simulink model "ce4951txrcv"  (R2020b)
settings: Solver=VariableStepAuto  StartTime=0.0  StopTime=32  RelTol=1e-3
libraries: simulink_extras x11, dspsrcs4 x1
settings Model: Creator=Andy  LastModifiedBy=Andy

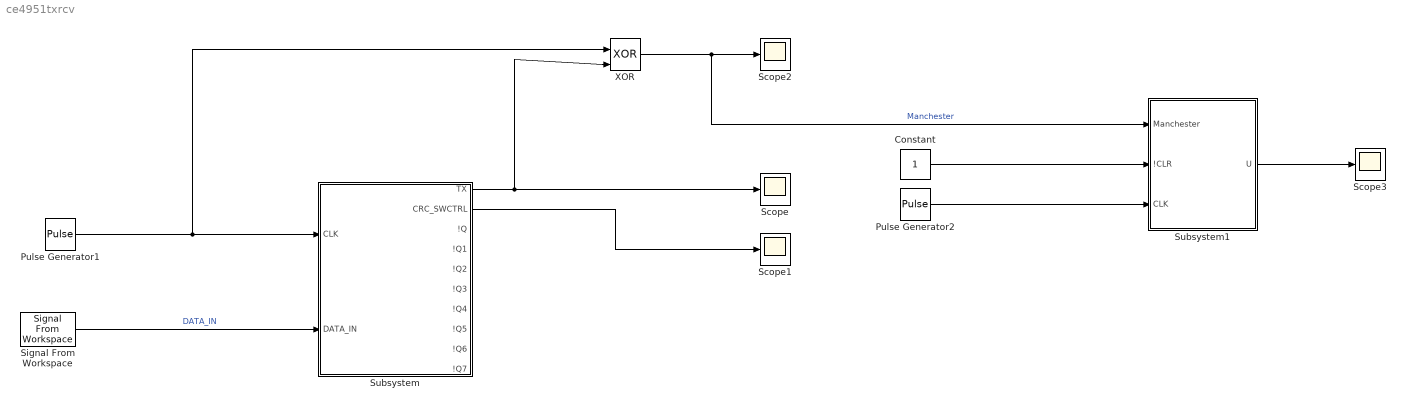
== system ce4951txrcv ==
  Constant : Constant
  Pulse Generator1 : DiscretePulseGenerator  PulseType=Time based  Period=1  PulseWidth=50
  Pulse Generator2 : DiscretePulseGenerator  PulseType=Time based  Period=0.5  PulseWidth=50
  Scope{,1..3} (4 alike) : Scope
  Signal From Workspace : dspsrcs4/Signal From Workspace  X=[0 1 0 0 0 0 0 1 0 1 0 0 0 0 1 0 0 1 0 0 0 0 1 1 0 0 0 0 0 0 0 0]  Ts=1  nsamps=1  OutputAfterFinalValue=Setting to zero  ignoreOrWarnInputAndFrameLengths=off  OutputFrames=off
  Subsystem : Subsystem
  Subsystem1 : Subsystem
  XOR : Logic  Operator=XOR  IconShape=distinctive  AllPortsSameDT=off  OutDataTypeStr=boolean
  wires:
  Subsystem/2(CRC_SWCTRL) -> Scope1/1
  XOR/1 -> Subsystem1/1(Manchester), Scope2/1  "Manchester"
  Signal From Workspace/1 -> Subsystem/2(DATA_IN)  "DATA_IN"
  Subsystem/1(TX) -> XOR/2, Scope/1
  Pulse Generator1/1 -> XOR/1, Subsystem/1(CLK)
  Pulse Generator2/1 -> Subsystem1/3(CLK)
  Constant/1 -> Subsystem1/2(!CLR)
  Subsystem1/1(U) -> Scope3/1

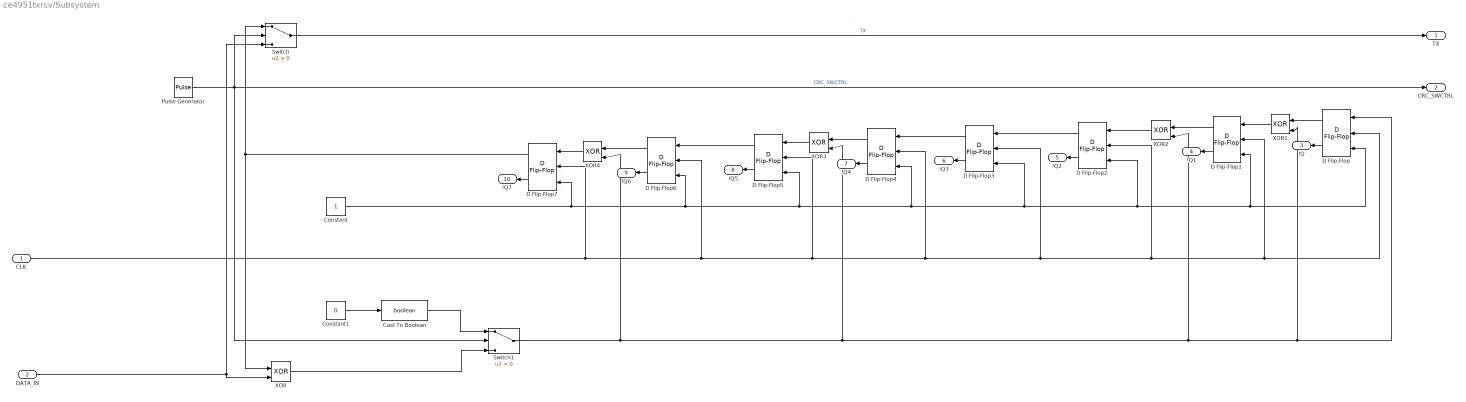
== system ce4951txrcv/Subsystem ==
  CLK : Inport
  DATA_IN : Inport  Port=2
  Cast To Boolean : DataTypeConversion  OutDataTypeStr=boolean
  Constant : Constant
  Constant1 : Constant  Value=0
  D Flip-Flop{,1..7} (8 alike) : simulink_extras/Flip Flops/D Flip-Flop
  Pulse Generator : DiscretePulseGenerator  PulseType=Time based  Period=32  PulseWidth=25  PhaseDelay=24
  Switch : Switch  Criteria=u2 > Threshold
  Switch1 : Switch  Criteria=u2 > Threshold
  XOR{,1..4} (5 alike) : Logic  Operator=XOR  IconShape=distinctive  AllPortsSameDT=off  OutDataTypeStr=boolean
  TX : Outport
  CRC_SWCTRL : Outport  Port=2
  !Q : Outport  Port=3
  !Q1 : Outport  Port=4
  !Q2 : Outport  Port=5
  !Q3 : Outport  Port=6
  !Q4 : Outport  Port=7
  !Q5 : Outport  Port=8
  !Q6 : Outport  Port=9
  !Q7 : Outport  Port=10
  wires:
  XOR1/1 -> D Flip-Flop1/1
  D Flip-Flop2/2 -> !Q2/1
  Constant1/1 -> Cast To Boolean/1
  D Flip-Flop4/2 -> !Q4/1
  CLK/1 -> D Flip-Flop6/2, D Flip-Flop5/2, D Flip-Flop4/2, D Flip-Flop3/2, D Flip-Flop2/2, D Flip-Flop1/2, D Flip-Flop/2, D Flip-Flop7/2
  D Flip-Flop7/1 -> Switch/1, XOR/1
  D Flip-Flop1/1 -> XOR2/1
  Constant/1 -> D Flip-Flop5/3, D Flip-Flop4/3, D Flip-Flop3/3, D Flip-Flop2/3, D Flip-Flop1/3, D Flip-Flop/3, D Flip-Flop6/3, D Flip-Flop7/3
  Switch/1 -> TX/1  "TX"
  D Flip-Flop5/1 -> D Flip-Flop6/1
  Switch1/1 -> XOR4/2, XOR2/2, XOR1/2, D Flip-Flop/1, XOR3/2
  Pulse Generator/1 -> CRC_SWCTRL/1, Switch1/2, Switch/2  "CRC_SWCTRL"
  XOR2/1 -> D Flip-Flop2/1
  XOR3/1 -> D Flip-Flop5/1
  D Flip-Flop6/2 -> !Q6/1
  DATA_IN/1 -> Switch/3, XOR/2
  D Flip-Flop3/1 -> D Flip-Flop4/1
  D Flip-Flop5/2 -> !Q5/1
  Cast To Boolean/1 -> Switch1/1
  D Flip-Flop2/1 -> D Flip-Flop3/1
  D Flip-Flop/1 -> XOR1/1
  XOR/1 -> Switch1/3
  D Flip-Flop4/1 -> XOR3/1
  D Flip-Flop3/2 -> !Q3/1
  D Flip-Flop6/1 -> XOR4/1
  D Flip-Flop/2 -> !Q/1
  XOR4/1 -> D Flip-Flop7/1
  D Flip-Flop7/2 -> !Q7/1
  D Flip-Flop1/2 -> !Q1/1

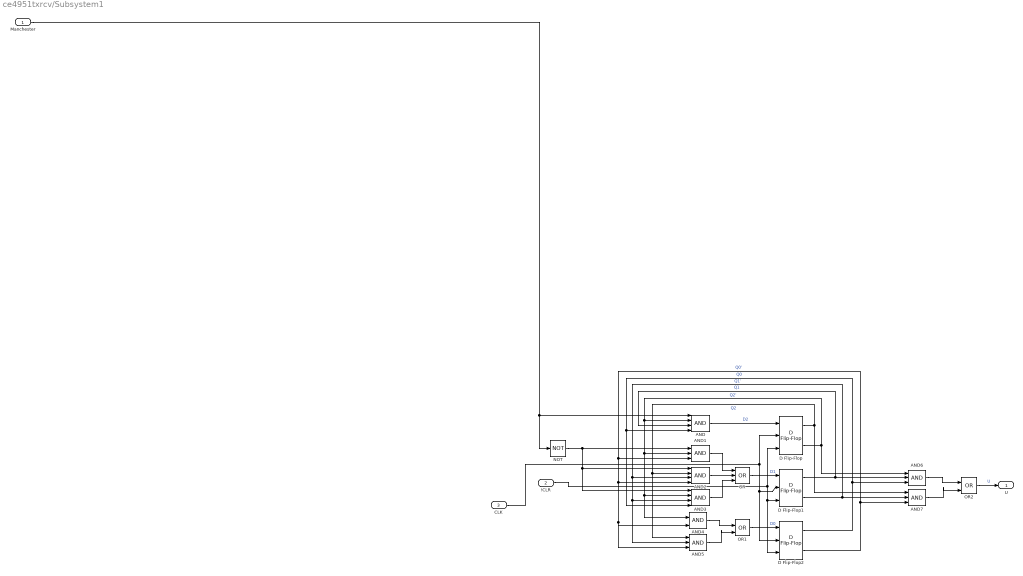
== system ce4951txrcv/Subsystem1 ==
  Manchester : Inport
  !CLR : Inport  Port=2
  CLK : Inport  Port=3
  AND : Logic  Inputs=4  IconShape=distinctive  AllPortsSameDT=off  OutDataTypeStr=boolean
  AND{1,5..7} (4 alike) : Logic  Inputs=3  IconShape=distinctive  AllPortsSameDT=off  OutDataTypeStr=boolean
  AND2 : Logic  Inputs=4  IconShape=distinctive  AllPortsSameDT=off  OutDataTypeStr=boolean
  AND3 : Logic  Inputs=4  IconShape=distinctive  AllPortsSameDT=off  OutDataTypeStr=boolean
  AND4 : Logic  IconShape=distinctive  AllPortsSameDT=off  OutDataTypeStr=boolean
  D Flip-Flop : simulink_extras/Flip Flops/D Flip-Flop
  D Flip-Flop1 : simulink_extras/Flip Flops/D Flip-Flop
  D Flip-Flop2 : simulink_extras/Flip Flops/D Flip-Flop
  NOT : Logic  Operator=NOT  IconShape=distinctive  AllPortsSameDT=off  OutDataTypeStr=boolean
  OR : Logic  Operator=OR  Inputs=3  IconShape=distinctive  AllPortsSameDT=off  OutDataTypeStr=boolean
  OR1 : Logic  Operator=OR  IconShape=distinctive  AllPortsSameDT=off  OutDataTypeStr=boolean
  OR2 : Logic  Operator=OR  IconShape=distinctive  AllPortsSameDT=off  OutDataTypeStr=boolean
  U : Outport
  wires:
  OR/1 -> D Flip-Flop1/1  "D1"
  D Flip-Flop2/1 -> AND6/3, AND/4, AND3/4  "Q0"
  !CLR/1 -> D Flip-Flop1/3, D Flip-Flop2/3, D Flip-Flop/3
  AND/1 -> D Flip-Flop/1  "D2"
  NOT/1 -> AND3/1, AND2/1, AND1/1
  D Flip-Flop1/2 -> AND7/2, AND2/3, AND3/3, AND5/2  "Q1'"
  AND2/1 -> OR/2
  AND1/1 -> OR/1
  AND3/1 -> OR/3
  Manchester/1 -> NOT/1, AND/1
  D Flip-Flop2/2 -> AND7/3, AND1/3, AND2/4, AND4/2, AND5/3  "Q0'"
  CLK/1 -> D Flip-Flop/2, D Flip-Flop2/2, D Flip-Flop1/2
  D Flip-Flop/2 -> AND/2, AND1/2, AND3/2, AND4/1, AND6/1  "Q2'"
  AND4/1 -> OR1/1
  D Flip-Flop1/1 -> AND6/2, AND/3  "Q1"
  D Flip-Flop/1 -> AND7/1, AND2/2, AND5/1  "Q2"
  AND5/1 -> OR1/2
  OR1/1 -> D Flip-Flop2/1  "D0"
  OR2/1 -> U/1  "U"
  AND6/1 -> OR2/1
  AND7/1 -> OR2/2
